simulink model "PIRControllerTest"  (R2022b)
settings: Solver=VariableStepAuto  StartTime=0.0  StopTime=30  RelTol=1e-3
undefined symbols (not defined in the file or in its folder): DiscIntNeverNeededParam, Krc, Krc2, magnitude, omegaC, omegaC2, omegaRes, omegaRes2, ts_spd_sec
libraries: simulink x6, slpidlib x1
settings Model: Creator=E1394481  LastModifiedBy=E1394481
settings SolverCC: ZeroCrossAlgorithm=Adaptive
settings DebuggingCC: IgnoredZcDiagnostic=none

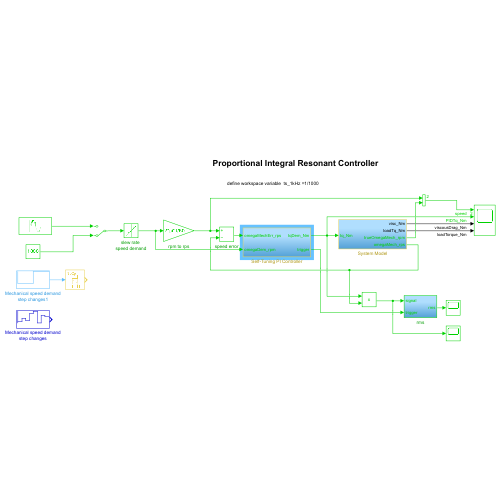
[thumbnail: Simulink's stored preview of the top-level diagram]
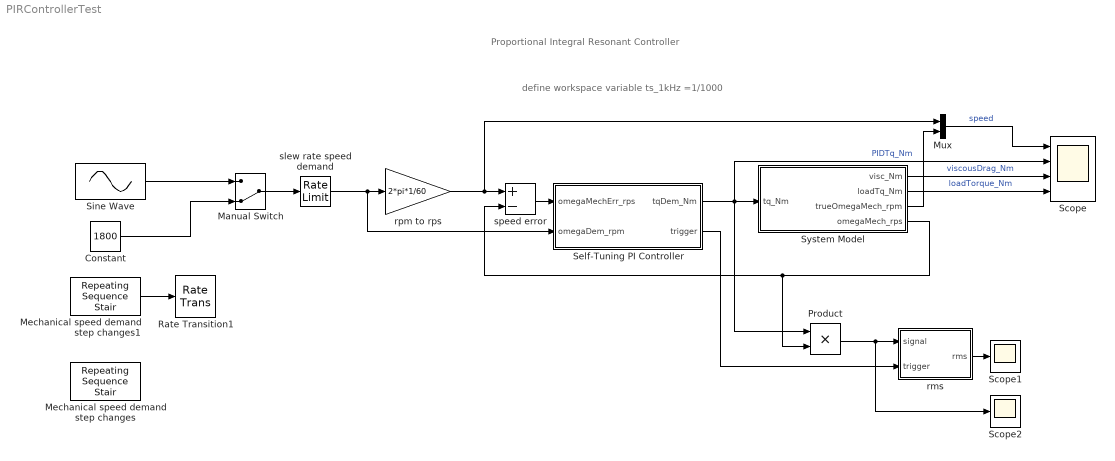
== system PIRControllerTest ==
  note: define workspace variable ts_1kHz =1/1000
  note: Proportional Integral Resonant Controller
  Constant : Constant  Value=1800  SampleTime=ts_spd_sec
  Manual Switch : ManualSwitch  CurrentSetting=0
  Mechanical speed demand step changes : simulink/Sources/Repeating Sequence Stair  OutValues=[1800 3600 2200 6000 7200 1200 5000 4500].'  tsamp=10  OutMin=[]  OutMax=[]  OutDataTypeStr=double  OutputDataTypeScalingMode=double  OutDataType=fixdt(0,8)  ConRadixGroup=Best Precision: Vector-wise  OutScaling=2^-12
  Mechanical speed demand step changes1 : simulink/Sources/Repeating Sequence Stair  OutValues=[1800 2200]  tsamp=200  OutMin=[]  OutMax=[]  OutDataTypeStr=double  OutputDataTypeScalingMode=double  OutDataType=fixdt(0,8)  ConRadixGroup=Best Precision: Vector-wise  OutScaling=2^-12
  Mux : Mux  Inputs=2
  Product : Product
  Rate Transition1 : RateTransition  OutPortSampleTime=ts_spd_sec
  Scope : Scope  NumInputPorts=4
  Scope1 : Scope
  Scope2 : Scope
  Self-Tuning PI Controller : Subsystem
  Sine Wave : Sin  Amplitude=1000  Bias=4500  Frequency=0.5  SampleTime=ts_spd_sec
  System Model : Subsystem
  rms : Subsystem
  rpm to rps : Gain  Gain=2*pi*1/60
  slew rate speed demand : RateLimiter  RisingSlewLimit=6500  FallingSlewLimit=-6500  SampleTimeMode=inherited
  speed error : Sum  Inputs=+-
  wires:
  rpm to rps/1 -> speed error/1, Mux/1
  speed error/1 -> Self-Tuning PI Controller/1(omegaMechErr_rps)
  System Model/4(omegaMech_rps) -> speed error/2, Product/2
  Self-Tuning PI Controller/1(tqDem_Nm) -> System Model/1(tq_Nm), Product/1, Scope/2  "PIDTq_Nm"
  Mux/1 -> Scope/1  "speed"
  slew rate speed demand/1 -> Self-Tuning PI Controller/2(omegaDem_rpm), rpm to rps/1
  System Model/1(visc_Nm) -> Scope/3  "viscousDrag_Nm"
  System Model/2(loadTq_Nm) -> Scope/4  "loadTorque_Nm"
  Manual Switch/1 -> slew rate speed demand/1
  System Model/3(trueOmegaMech_rpm) -> Mux/2
  rms/1(rms) -> Scope1/1
  Product/1 -> Scope2/1, rms/1(signal)
  Sine Wave/1 -> Manual Switch/1
  Mechanical speed demand step changes1/1 -> Rate Transition1/1
  Constant/1 -> Manual Switch/2
  Self-Tuning PI Controller/2(trigger) -> rms/2(trigger)

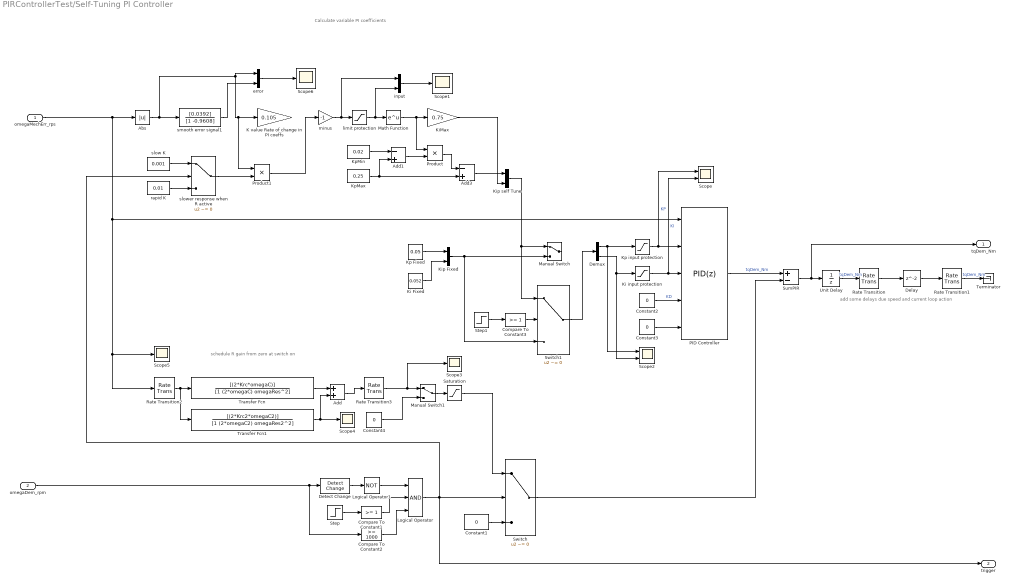
== system PIRControllerTest/Self-Tuning PI Controller ==
  note: schedule R gain from zero at switch on
  note: add some delays due speed and current loop action
  note: Calculate variable PI coefficients
  omegaMechErr_rps : Inport
  omegaDem_rpm : Inport  Port=2
  Abs : Abs  SaturateOnIntegerOverflow=off
  Add : Sum
  Add1 : Sum  Inputs=-+
  Add3 : Sum  Inputs=-+
  Compare To Constant1 : simulink/Logic and Bit Operations/Compare To Constant  relop=>=  const=1  OutDataTypeStr=boolean
  Compare To Constant2 : simulink/Logic and Bit Operations/Compare To Constant  relop=>=  const=1000  OutDataTypeStr=boolean
  Compare To Constant3 : simulink/Logic and Bit Operations/Compare To Constant  relop=>=  const=1  OutDataTypeStr=boolean
  Constant{1..4} (4 alike) : Constant  Value=0  SampleTime=ts_spd_sec
  Delay : Delay  SampleTime=1/8000
  Demux : Demux  Outputs=2
  Detect Change : simulink/Logic and Bit Operations/Detect Change  vinit=0  OutDataTypeStr=boolean
  K value Rate of change in PI coeffs : Gain  Gain=0.105
  Ki Fixed : Constant  Value=0.052  SampleTime=ts_spd_sec
  Ki input protection : Saturate  UpperLimit=2  LowerLimit=0
  KiMax : Gain  Gain=0.75
  Kip Fixed : Mux  Inputs=2
  Kip self Tune : Mux  Inputs=2
  Kp Fixed : Constant  Value=0.05  SampleTime=ts_spd_sec
  Kp input protection : Saturate  UpperLimit=2  LowerLimit=0
  KpMax : Constant  Value=0.25  SampleTime=ts_spd_sec
  KpMin : Constant  Value=0.02  SampleTime=ts_spd_sec
  Logical Operator : Logic  Inputs=3  AllPortsSameDT=off  OutDataTypeStr=boolean
  Logical Operator1 : Logic  Operator=NOT  AllPortsSameDT=off  OutDataTypeStr=boolean
  Manual Switch : ManualSwitch
  Manual Switch1 : ManualSwitch
  Math Function : Math
  PID Controller : slpidlib/PID Controller  Controller=PID  Form=Parallel  TimeDomain=Discrete-time  UseExternalTs=off  SampleTime=ts_spd_sec  IntegratorMethod=Forward Euler  FilterMethod=Forward Euler  ControllerParametersSource=external  P=0.01  I=0.01  UseKiTs=off  D=0  N=100  UseFilter=on  TunerSelectOption=Transfer Function Based (PID Tuner App)  InitialConditionSource=internal  InitialConditionForIntegrator=0  InitialConditionForFilter=0  DifferentiatorICPrevScaledInput=0  ExternalReset=none  TrackingMode=off  Kt=1  LimitOutput=on  SatLimitsSource=internal  UpperSaturationLimit=9.25  LowerSaturationLimit=-9.25  LinearizeAsGain=on  AntiWindupMode=clamping  Kb=1  LimitIntegrator=on  UpperIntegratorSaturationLimit=8.5  LowerIntegratorSaturationLimit=-8.5  RndMeth=Nearest  POutMin=[]  POutMax=[]  IOutMin=[]  IOutMax=[]  DOutMin=[]  DOutMax=[]  NOutMin=[]  NOutMax=[]  SumOutMin=[]  SumOutMax=[]  SaturationOutMin=[]  SaturationOutMax=[]  PParamMin=[]  PParamMax=[]  IParamMin=[]  IParamMax=[]  DParamMin=[]  DParamMax=[]  NParamMin=[]  NParamMax=[]  KbParamMin=[]  KbParamMax=[]  KtParamMin=[]  KtParamMax=[]  KbOutMin=[]  KbOutMax=[]  KtOutMin=[]  KtOutMax=[]  IntegratorOutMin=[]  IntegratorOutMax=[]  FilterOutMin=[]  FilterOutMax=[]  SumI1OutMin=[]  SumI1OutMax=[]  SumI2OutMin=[]  SumI2OutMax=[]  SumI3OutMin=[]  SumI3OutMax=[]  SumI4OutMin=[]  SumI4OutMax=[]  SumDOutMin=[]  SumDOutMax=[]  DifferentiatorOutMin=[]  DifferentiatorOutMax=[]  FilterDiffOutCoefMin=[]  FilterDiffOutCoefMax=[]  ReciprocalOutMin=[]  ReciprocalOutMax=[]  SumDenOutMin=[]  SumDenOutMax=[]  SumNumOutMin=[]  SumNumOutMax=[]  DivideOutMin=[]  DivideOutMax=[]  UdiffTsProdOutMin=[]  UdiffTsProdOutMax=[]  NTsProdOutMin=[]  NTsProdOutMax=[]  UintegralTsProdOutMin=[]  UintegralTsProdOutMax=[]  UngainTsProdOutMin=[]  UngainTsProdOutMax=[]  ClampingZeroOutDataTypeStr=Inherit: Inherit via back propagation  ClampingZeroOutMin=[]  ClampingZeroOutMax=[]  FilterDenConstantOutDataTypeStr=Inherit: Inherit via back propagation  FilterDenConstantOutMin=[]  FilterDenConstantOutMax=[]  PCopyOutDataTypeStr=Inherit: Inherit via back propagation  PCopyOutMin=[]  PCopyOutMax=[]  NCopyOutDataTypeStr=Inherit: Inherit via back propagation  NCopyOutMin=[]  NCopyOutMax=[]  IntegratorContinuousStateAttributes=''  IntegratorStateMustResolveToSignalObject=off  IntegratorRTWStateStorageClass=Auto  FilterContinuousStateAttributes=''  FilterStateMustResolveToSignalObject=off  FilterRTWStateStorageClass=Auto  ParallelPVariant=ExternalParameters  IdealPVariant=Disabled  IVariant=ExternalParameters  DVariant=ExternalParameters  IntegratorVariant=Discrete  SatVariant=Enabled  AWVariant=DiscClampingParallel  PCopyVariant=Disabled  TRVariant=Disabled  FdbkBlocksVariant=Forward  IdealPFdbkVariant=Disabled  SatFdbkVariant=Disabled  DerivativeFilterVariant=ForwardEulerFilter  NVariant=ExternalParameters  NCopyVariant=Disabled  FilterICVariant=InternalICsFilter  IntegratorICVariant=InternalICs  ExternalResetVariant=Disabled  TRSumVariant=Passthrough  SumFdbkVariant=Disabled  SumVariant=Sum_PID  TsampFilterVariant=InternalTs  TsampNgainVariant=Passthrough  TsampIntegralVariant=Passthrough  ExternalSaturationOutDataTypeStr=Inherit: Same as second input
  Product : Product
  Product1 : Product
  Rate Transition{,1..3} (4 alike) : RateTransition
  Saturation : Saturate  UpperLimit=2  LowerLimit=-2
  Scope : Scope  NumInputPorts=2
  Scope{1,3..6} (5 alike) : Scope
  Scope2 : Scope  NumInputPorts=2
  Step : Step  Time=20  SampleTime=ts_spd_sec
  Step1 : Step  Time=15  SampleTime=ts_spd_sec
  SumPIR : Sum  Inputs=+-
  Switch : Switch  Criteria=u2 ~= 0  SaturateOnIntegerOverflow=off  InputSameDT=off
  Switch1 : Switch  Criteria=u2 ~= 0  SaturateOnIntegerOverflow=off  InputSameDT=off
  Terminator : Terminator
  Transfer Fcn : TransferFcn  Numerator=[(2*Krc*omegaC)]  Denominator=[1 (2*omegaC) omegaRes^2]
  Transfer Fcn1 : TransferFcn  Numerator=[(2*Krc2*omegaC2)]  Denominator=[1 (2*omegaC2) omegaRes2^2]
  Unit Delay : UnitDelay  SampleTime=ts_spd_sec  HasFrameUpgradeWarning=on
  error : Mux  Inputs=2
  input : Mux  Inputs=2
  limit protection : Saturate  UpperLimit=0  LowerLimit=-100
  minus : Gain  Gain=-1
  rapid K : Constant  Value=0.01  SampleTime=ts_spd_sec
  slow K : Constant  Value=0.001  SampleTime=ts_spd_sec
  slower response when R active : Switch  Criteria=u2 ~= 0  SaturateOnIntegerOverflow=off  InputSameDT=off
  smooth error signal1 : DiscreteFilter  Numerator=[0.0392]  Denominator=[1 -0.9608]
  tqDem_Nm : Outport
  trigger : Outport  Port=2
  wires:
  Unit Delay/1 -> Rate Transition/1  "tqDem_Nm"
  Constant2/1 -> PID Controller/4  "KD"
  Constant3/1 -> PID Controller/5
  Math Function/1 -> Product/1, KiMax/1
  KiMax/1 -> Kip self Tune/2
  Add1/1 -> Product/2
  Product/1 -> Add3/1
  Add3/1 -> Kip self Tune/1
  limit protection/1 -> input/2, Math Function/1
  KpMax/1 -> Add1/2, Add3/2
  Ki input protection/1 -> Scope/2, PID Controller/3  "KI"
  Kp input protection/1 -> Scope/1, PID Controller/2  "KP"
  Rate Transition/1 -> Delay/1
  Delay/1 -> Rate Transition1/1
  PID Controller/1 -> SumPIR/1  "tqDem_Nm"
  minus/1 -> input/1, limit protection/1
  KpMin/1 -> Add1/1
  Abs/1 -> K value Rate of change in PI coeffs/1, Product1/1, error/1, smooth error signal1/1
  Kp Fixed/1 -> Kip Fixed/1
  Ki Fixed/1 -> Kip Fixed/2
  Kip self Tune/1 -> Switch1/1, Manual Switch/1
  Kip Fixed/1 -> Manual Switch/2, Switch1/3
  Demux/2 -> Ki input protection/1, Scope2/2
  Demux/1 -> Scope2/1, Kp input protection/1
  SumPIR/1 -> tqDem_Nm/1, Unit Delay/1
  Rate Transition2/1 -> Transfer Fcn1/1, Transfer Fcn/1
  Rate Transition3/1 -> Scope3/1, Manual Switch1/1
  Constant1/1 -> Switch/3
  Switch/1 -> SumPIR/2
  Step1/1 -> Compare To Constant3/1
  omegaDem_rpm/1 -> Detect Change/1, Compare To Constant2/1
  Saturation/1 -> Switch/1
  Constant4/1 -> Manual Switch1/2
  Logical Operator1/1 -> Logical Operator/1
  Step/1 -> Compare To Constant1/1
  Compare To Constant1/1 -> Logical Operator/2
  Compare To Constant2/1 -> Logical Operator/3
  Compare To Constant3/1 -> Switch1/2
  omegaMechErr_rps/1 -> Abs/1, PID Controller/1, Rate Transition2/1, Scope5/1
  Manual Switch1/1 -> Saturation/1
  Logical Operator/1 -> Switch/2, trigger/1, slower response when R active/2
  Rate Transition1/1 -> Terminator/1  "tqDem_Nm"
  rapid K/1 -> slower response when R active/3
  Product1/1 -> minus/1
  slower response when R active/1 -> Product1/2
  Switch1/1 -> Demux/1
  Detect Change/1 -> Logical Operator1/1
  Transfer Fcn1/1 -> Scope4/1, Add/2
  Transfer Fcn/1 -> Add/1
  slow K/1 -> slower response when R active/1
  error/1 -> Scope6/1
  smooth error signal1/1 -> error/2
  input/1 -> Scope1/1
  Add/1 -> Rate Transition3/1

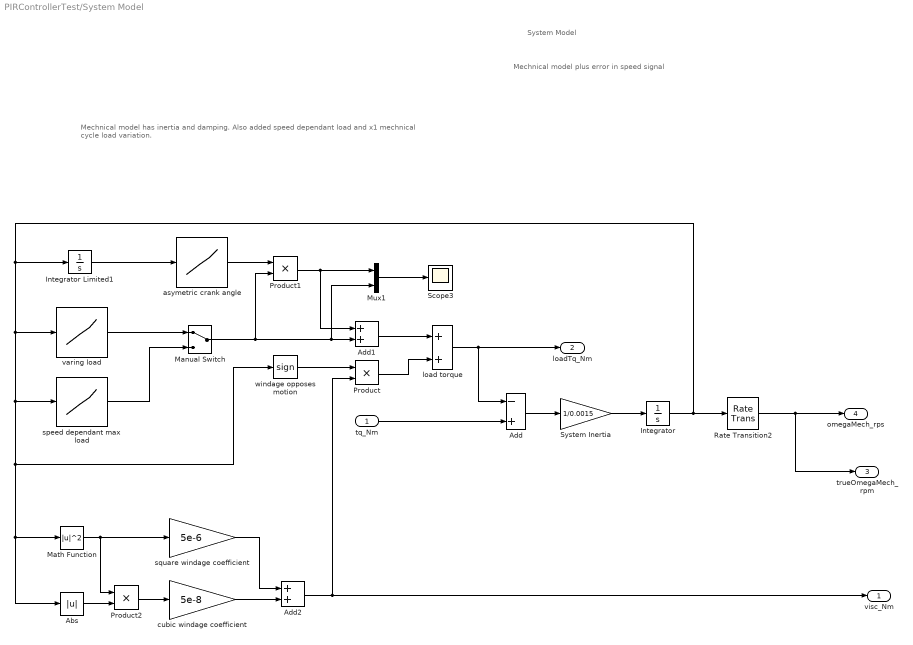
== system PIRControllerTest/System Model ==
  note: Mechnical model has inertia and damping. Also added speed dependant load and x1 mechnical cycle load variation.
  note: Mechnical model plus error in speed signal
  note: System Model
  tq_Nm : Inport
  Abs : Abs  SaturateOnIntegerOverflow=off
  Add : Sum  Inputs=-+
  Add1 : Sum
  Add2 : Sum
  Integrator : Integrator
  Integrator Limited1 : Integrator  UpperSaturationLimit=1  LowerSaturationLimit=0  WrapState=on
  Manual Switch : ManualSwitch
  Math Function : Math  Operator=magnitude^2
  Mux1 : Mux  Inputs=2
  Product : Product
  Product1 : Product
  Product2 : Product
  Rate Transition2 : RateTransition  OutPortSampleTime=ts_spd_sec
  Scope3 : Scope
  System Inertia : Gain  Gain=1/0.0015
  asymetric crank angle : Lookup_n-D  NumberOfTableDimensions=1  BreakpointsForDimension1="[-1 -0.8 -0.7    0       0.32   0.4  0.45 0.5  0.6   0.7  1]*pi"  BeginIndexSearchUsingPreviousIndexResult=on  Table="[0   0   0.01  0.02   0.05   0.1   0.3   0.3   0.2   0.1   0]"  ExtrapMethod=Clip  UseLastTableValue=on  ApplyFullPrecisionForLinearInterpolation=on  InternalRulePriority=Speed  RndMeth=Simplest
  cubic windage coefficient : Gain  Gain=5e-8
  load torque : Sum
  speed dependant max load : Lookup_n-D  NumberOfTableDimensions=1  BreakpointsForDimension1=[-100 0 100 1000 1200 2000 3000 4000 5000 6000 7000 8000]*2*pi*1/60  BeginIndexSearchUsingPreviousIndexResult=on  Table=[0 0 7 3 6 4 3 4 5 6 7 8] *0 +4  ExtrapMethod=Clip  UseLastTableValue=on  ApplyFullPrecisionForLinearInterpolation=on  InternalRulePriority=Speed  RndMeth=Simplest
  square windage coefficient : Gain  Gain=5e-6
  "varing load " : Lookup_n-D  NumberOfTableDimensions=1  BreakpointsForDimension1=[-100 0 100 1000 1600 1700 1800 2000 3000 4000 5000 6000 7000 8000]*2*pi*1/60  BeginIndexSearchUsingPreviousIndexResult=on  Table=[0 0 0.1 1 5 6 9 6 8 7 6 5 4 3] *0.75  ExtrapMethod=Clip  UseLastTableValue=on  ApplyFullPrecisionForLinearInterpolation=on  InternalRulePriority=Speed  RndMeth=Simplest
  windage opposes motion : Signum
  visc_Nm : Outport
  loadTq_Nm : Outport  Port=2
  trueOmegaMech_rpm : Outport  Port=3
  omegaMech_rps : Outport  Port=4
  wires:
  System Inertia/1 -> Integrator/1
  Math Function/1 -> Product2/1, square windage coefficient/1
  Add2/1 -> Product/2, visc_Nm/1
  windage opposes motion/1 -> Product/1
  Integrator Limited1/1 -> asymetric crank angle/1
  asymetric crank angle/1 -> Product1/1
  Manual Switch/1 -> Product1/2, Add1/2, Mux1/2
  tq_Nm/1 -> Add/2
  Product1/1 -> Mux1/1, Add1/1
  Product2/1 -> cubic windage coefficient/1
  square windage coefficient/1 -> Add2/1
  cubic windage coefficient/1 -> Add2/2
  Abs/1 -> Product2/2
  Integrator/1 -> Rate Transition2/1, Integrator Limited1/1, Abs/1, Math Function/1, windage opposes motion/1, speed dependant max load/1, "varing load "/1
  Rate Transition2/1 -> trueOmegaMech_rpm/1, omegaMech_rps/1
  Mux1/1 -> Scope3/1
  "varing load "/1 -> Manual Switch/1
  speed dependant max load/1 -> Manual Switch/2
  load torque/1 -> loadTq_Nm/1, Add/1
  Add1/1 -> load torque/1
  Product/1 -> load torque/2
  Add/1 -> System Inertia/1

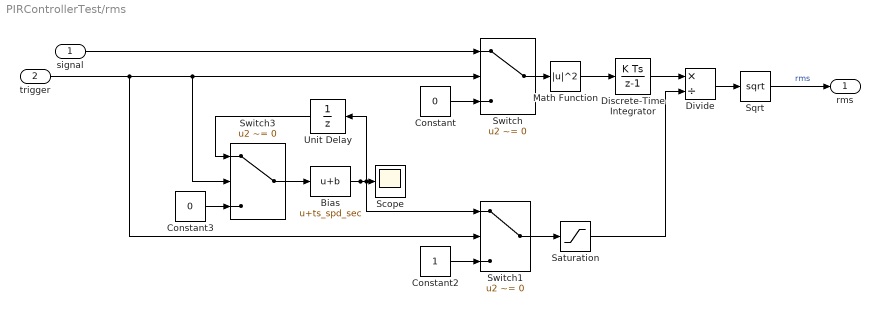
== system PIRControllerTest/rms ==
  signal : Inport
  trigger : Inport  Port=2
  Bias : Bias  Bias=ts_spd_sec  SaturateOnIntegerOverflow=off
  Constant : Constant  Value=0
  Constant2 : Constant
  Constant3 : Constant  Value=0
  Discrete-Time Integrator : DiscreteIntegrator  SampleTime=-1  ICPrevOutput=DiscIntNeverNeededParam  ICPrevScaledInput=DiscIntNeverNeededParam
  Divide : Product  Inputs=*/
  Math Function : Math  Operator=magnitude^2
  Saturation : Saturate  UpperLimit=inf  LowerLimit=ts_spd_sec
  Scope : Scope
  Sqrt : Sqrt
  Switch : Switch  Criteria=u2 ~= 0  SaturateOnIntegerOverflow=off  InputSameDT=off
  Switch1 : Switch  Criteria=u2 ~= 0  SaturateOnIntegerOverflow=off  InputSameDT=off
  Switch3 : Switch  Criteria=u2 ~= 0  SaturateOnIntegerOverflow=off  InputSameDT=off
  Unit Delay : UnitDelay  SampleTime=-1  HasFrameUpgradeWarning=on
  rms : Outport
  wires:
  Divide/1 -> Sqrt/1
  Switch/1 -> Math Function/1
  Sqrt/1 -> rms/1  "rms"
  Math Function/1 -> Discrete-Time Integrator/1
  Discrete-Time Integrator/1 -> Divide/1
  Saturation/1 -> Divide/2
  signal/1 -> Switch/1
  trigger/1 -> Switch1/2, Switch3/2, Switch/2
  Constant/1 -> Switch/3
  Bias/1 -> Switch1/1, Unit Delay/1, Scope/1
  Constant2/1 -> Switch1/3
  Switch1/1 -> Saturation/1
  Switch3/1 -> Bias/1
  Unit Delay/1 -> Switch3/1
  Constant3/1 -> Switch3/3
